simulink model "sxem_sravn"  (R2015b)
settings: Solver=VariableStepAuto  StartTime=0.0  StopTime=1  RelTol=1e-3
settings Model: Creator=hohotulca  LastModifiedBy=hohotulca

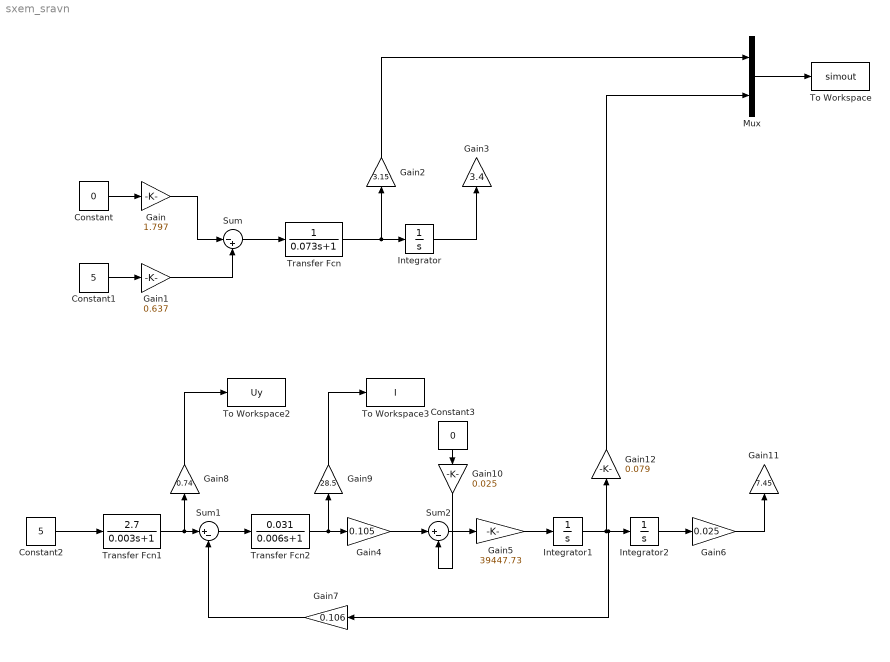
== system sxem_sravn ==
  Constant : Constant  Value=0
  Constant1 : Constant  Value=5
  Constant2 : Constant  Value=5
  Constant3 : Constant  Value=0
  Gain : Gain  Gain=1.797
  Gain1 : Gain  Gain=0.637
  Gain10 : Gain  Gain=0.025
  Gain11 : Gain  Gain=7.45
  Gain12 : Gain  Gain=0.079
  Gain2 : Gain  Gain=3.15
  Gain3 : Gain  Gain=3.4
  Gain4 : Gain  Gain=0.105
  Gain5 : Gain  Gain=39447.73
  Gain6 : Gain  Gain=0.025
  Gain7 : Gain  Gain=0.106
  Gain8 : Gain  Gain=0.74
  Gain9 : Gain  Gain=28.5
  Integrator : Integrator
  Integrator1 : Integrator
  Integrator2 : Integrator
  Mux : Mux  Inputs=2
  Sum : Sum  Inputs=|-+
  Sum1 : Sum  Inputs=|+-
  Sum2 : Sum  Inputs=|+-
  To Workspace : ToWorkspace  VariableName=simout  SaveFormat=Timeseries  SampleTime=-1
  To Workspace2 : ToWorkspace  VariableName=Uy  SaveFormat=Timeseries  SampleTime=-1
  To Workspace3 : ToWorkspace  VariableName=I  SaveFormat=Timeseries  SampleTime=-1
  Transfer Fcn : TransferFcn  Denominator=[0.073 1]
  Transfer Fcn1 : TransferFcn  Numerator=[2.7]  Denominator=[0.003 1]
  Transfer Fcn2 : TransferFcn  Numerator=[0.031]  Denominator=[0.006 1]
  wires:
  Constant/1 -> Gain/1
  Constant1/1 -> Gain1/1
  Gain1/1 -> Sum/2
  Gain/1 -> Sum/1
  Sum/1 -> Transfer Fcn/1
  Transfer Fcn/1 -> Gain2/1, Integrator/1
  Integrator/1 -> Gain3/1
  Constant2/1 -> Transfer Fcn1/1
  Transfer Fcn1/1 -> Gain8/1, Sum1/1
  Sum1/1 -> Transfer Fcn2/1
  Transfer Fcn2/1 -> Gain9/1, Gain4/1
  Gain4/1 -> Sum2/1
  Sum2/1 -> Gain5/1
  Gain5/1 -> Integrator1/1
  Integrator1/1 -> Gain7/1, Integrator2/1, Gain12/1
  Integrator2/1 -> Gain6/1
  Gain7/1 -> Sum1/2
  Gain8/1 -> To Workspace2/1
  Gain9/1 -> To Workspace3/1
  Gain10/1 -> Sum2/2
  Constant3/1 -> Gain10/1
  Gain6/1 -> Gain11/1
  Gain2/1 -> Mux/1
  Gain12/1 -> Mux/2
  Mux/1 -> To Workspace/1
